simulink model "uplink_downlink"  (R2023a)
settings: Solver=VariableStepAuto  StartTime=0.0  StopTime=10  RelTol=1e-3
libraries: rfmathmodels2 x2, commdigbbndpm3 x2, commchan3 x1, commrandsrc3 x1, commsink2 x1
settings Model: Creator=ynsmr  LastModifiedBy=ynsmr

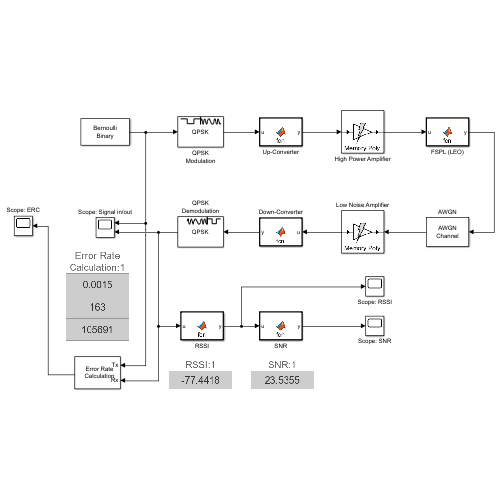
[thumbnail: Simulink's stored preview of the top-level diagram]
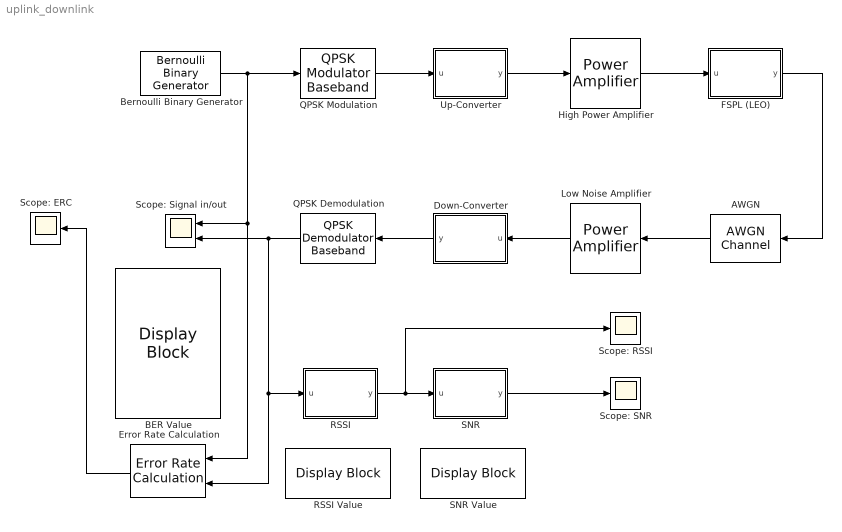
== system uplink_downlink ==
  AWGN : commchan3/AWGN Channel  LegacyMode=off  NoiseMethod="Signal to noise ratio  (SNR)"  noiseMode="Signal to noise ratio  (SNR)"  EbNo=10  EsNo=10  SNR=111  BitsPerSymbol=1  SignalPower=1  SamplesPerSymbol=1  SymbolPeriod=1  VarianceSource=Parameter  Variance=1  RandomStream=Global stream  Seed=67  SimulateUsing=Code generation
  BER Value : DisplayBlock  Transparency=1
  Bernoulli Binary Generator : commrandsrc3/Bernoulli Binary Generator  ProbabilityOfZero=0.5  SeedSource=Parameter  Seed=0  SampleTime=1/1e6  SamplesPerFrame=1  OutputDataType=double  SimulateUsing=Interpreted execution
  Down-Converter : MATLAB Function  TreatAsAtomicUnit=on
  Error Rate Calculation : commsink2/Error Rate Calculation  N=0  st_delay=0  cp_mode=Entire frame  subframe=[]  PMode=Port  WsName=ErrorVec  RsMode2=off  stop=off  numErr=100  maxBits=1e6
  FSPL (LEO) : MATLAB Function  TreatAsAtomicUnit=on
  High Power Amplifier : rfmathmodels2/Power Amplifier  ModelType=Memory polynomial  CoefficientMatrix=375  UnitDelay=1e-06  SamplesPerUnitDelay=1  SimulateUsing=Code generation
  Low Noise Amplifier : rfmathmodels2/Power Amplifier  ModelType=Memory polynomial  CoefficientMatrix=20  UnitDelay=1e-06  SamplesPerUnitDelay=1  SimulateUsing=Code generation
  QPSK Demodulation : commdigbbndpm3/QPSK Demodulator Baseband  OutType=Integer  DecType=Hard decision  VarSource=Dialog  Variance=1  Dec=Gray  Ph=pi/4  outDtype1=Inherit via internal rule  outDtype2=double  derotateFactorWordLen=16  derotateFactorDataTypeStr=Inherit: Same word length as input  derotateFactorLastDataTypeStr=Inherit: Same word length as input
  QPSK Modulation : commdigbbndpm3/QPSK Modulator Baseband  InType=Integer  Enc=Gray  Ph=pi/4  outDtype=double  outWordLen=16  outUDDataType=sfix(16)  outFracLenMode=Best precision  outFracLen=15  outDataTypeStr=double  outLastDataTypeStr=double
  RSSI : MATLAB Function  TreatAsAtomicUnit=on
  RSSI Value : DisplayBlock  Transparency=1
  SNR : MATLAB Function  TreatAsAtomicUnit=on
  SNR Value : DisplayBlock  Transparency=1
  Scope: ERC : Scope
  Scope: RSSI : Scope
  Scope: SNR : Scope
  Scope: Signal in/out : Scope  NumInputPorts=2
  Up-Converter : MATLAB Function  TreatAsAtomicUnit=on
  wires:
  SNR/1(y) -> Scope: SNR/1
  FSPL (LEO)/1(y) -> AWGN/1
  QPSK Demodulation/1 -> RSSI/1(u), Error Rate Calculation/2, Scope: Signal in/out/2
  Down-Converter/1(y) -> QPSK Demodulation/1
  QPSK Modulation/1 -> Up-Converter/1(u)
  Up-Converter/1(y) -> High Power Amplifier/1
  RSSI/1(y) -> Scope: RSSI/1, SNR/1(u)
  Bernoulli Binary Generator/1 -> QPSK Modulation/1, Error Rate Calculation/1, Scope: Signal in/out/1
  High Power Amplifier/1 -> FSPL (LEO)/1(u)
  Low Noise Amplifier/1 -> Down-Converter/1(u)
  AWGN/1 -> Low Noise Amplifier/1
  Error Rate Calculation/1 -> Scope: ERC/1

== matlab function uplink_downlink/RSSI ==
  data: u input; y output
function y = fcn(u)
P_TX = 40; % dBm (başlangıç gücü)
G_TX = 30; % dBi (antenn kazancı, PA_TX_Combined’da dahil)
G_RX = 20; % dBi (alıcı kazancı)
d = 500e3; % Mesafe (m)
f = 2e9; % Frekans (Hz)
c = 3e8; % Işık hızı
L_other = 5; % Diğer kayıplar (dB)
FSPL = 20*log10(d) + 20*log10(f) + 20*log10(4*pi/c);
signal_power = mean(abs(u).^2); % Kompleks sinyalin gücü
signal_power_dBm = 10*log10(signal_power*1000); % mW’a çevir
y = P_TX + G_TX + G_RX - FSPL - L_other + signal_power_dBm - 40; % RSSI (dBm)

== matlab function uplink_downlink/FSPL (LEO) ==
  data: u input; y output
function y = fcn(u)
d = 500e3; % Mesafe (m)
f = 2e9; % Frekans (Hz)
c = 3e8; % Işık hızı (m/s)
FSPL = 20*log10(d) + 20*log10(f) + 20*log10(4*pi/c); % dB
y = u / (10^(FSPL/20)); % Sinyali zayıflat

== matlab function uplink_downlink/Up-Converter ==
  data: u input; y output
function y = fcn(u)
% Giriş sinyali skaler veya vektör olabilir
fc = 12e9; % Taşıyıcı frekansı (2 GHz)
Ts = 1/1e6; % Örnekleme süresi (1 MHz, Bernoulli ile uyumlu)
persistent t; % Zamanı saklamak için kalıcı değişken
if isempty(t)
    t = 0; % Başlangıçta t=0
end
y = u .* exp(1j*2*pi*fc*t); % Sinyali RF’ye kaydır
t = t + Ts; % Zamanı bir örnek artır

== matlab function uplink_downlink/Down-Converter ==
  data: u input; y output
function y = fcn(u)
% Giriş sinyali skaler veya vektör olabilir
fc = 2e9; % Taşıyıcı frekansı (2 GHz)
Ts = 1/1e6; % Örnekleme süresi (1 MHz)
persistent t; % Zamanı saklamak için kalıcı değişken
if isempty(t)
    t = 0; % Başlangıçta t=0
end
y = u .* exp(-1j*2*pi*fc*t); % Sinyali baseband’e indir
t = t + Ts; % Zamanı bir örnek artır

== matlab function uplink_downlink/SNR ==
  data: u input; y output
function y = fcn(u)
k = 1.38e-23; % Boltzmann sabiti
T = 290; % Sıcaklık (K)
B = 10e6; % Bant genişliği (Hz)
NF = 3; % Gürültü faktörü (dB)
N_dBm = 10*log10(k*T*B*1000) + NF; % Gürültü gücü
y = u - N_dBm; % SNR (dB)
